simulink model "Pid"  (R2020b)
settings: Solver=VariableStepAuto  StartTime=0.0  StopTime=10.0  RelTol=1e-3
model workspace (MAT data in the model file):
  Ki = Simulink.Parameter
  Ki.Value = 50
  Ki.DataType = 'auto'
  Ki.Dimensions = [1 1]
  Kp = Simulink.Parameter
  Kp.Value = 600
  Kp.DataType = 'auto'
  Kp.Dimensions = [1 1]
settings Model: Creator=Lenovo  LastModifiedBy=Lenovo

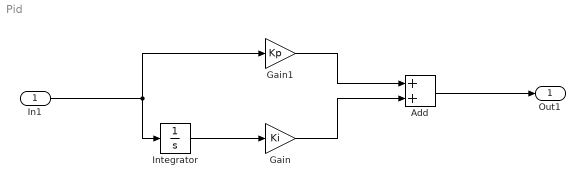
== system Pid ==
  In1 : Inport
  Add : Sum
  Gain : Gain  Gain=Ki
  Gain1 : Gain  Gain=Kp
  Integrator : Integrator
  Out1 : Outport
  wires:
  In1/1 -> Integrator/1, Gain1/1
  Integrator/1 -> Gain/1
  Gain1/1 -> Add/1
  Gain/1 -> Add/2
  Add/1 -> Out1/1
